simulink model "power_acvoltage"  (Simulink 6.0)
settings: Solver=VariableStepDiscrete  SolverMode=SingleTasking  StartTime=0.0  StopTime=888  MaxStep=1e-03  RelTol=1e-3  AbsTol=1e-6
libraries: powerlib x4
settings Model: Creator=patrice  LastModifiedBy=batserve  ExtModeTrigMode=oneshot  ExtModeArmWhenConnect=off  ExtModeAutoUpdateStatusClock=off
settings DataIOCC: LimitDataPoints=off  SignalLoggingName=sigsOut
settings OptimizationCC: BooleanDataType=off
settings DebuggingCC: SolverPrmCheckMsg=none
settings HardwareCC: TargetUnknown=on
settings RTWCC: TemplateMakefile=grt_unix.tmf

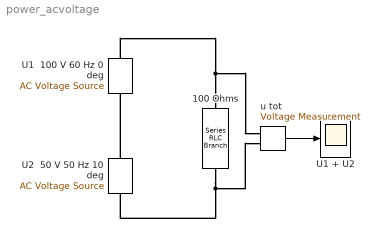
== system power_acvoltage ==
  100 Ohms : powerlib/Elements/Series RLC Branch  Orientation=down  PhysicalDomain=powersysdomain  SubClassName=unknown  PortType=p1  LConnTagsString=__new0  RConnTagsString=__new0  Resistance=100  Inductance=0  Capacitance=inf  Measurements=None
  U1  100 V 60 Hz 0 deg : powerlib/Electrical Sources/AC Voltage Source  Description=source block  Orientation=up  Amplitude=100  Phase=0  Frequency=60  SampleTime=0  Measurements=None
      settings: AttributesFormatString=\n
  U1 + U2 : Scope
      settings: TickLabels=on  TimeRange=0.5  YMin=-180  YMax=180  DataFormat=Array
  U2  50 V 50 Hz 10 deg : powerlib/Electrical Sources/AC Voltage Source  Description=source block  Orientation=up  Amplitude=50  Phase=10  Frequency=50  SampleTime=0  Measurements=None
      settings: AttributesFormatString=\n
  u tot : powerlib/Measurements/Voltage Measurement  Tag=PoWeRsYsTeMmEaSuReMeNt  PhasorSimulation=off  OutputType=Magnitude  PSBequivalent=0
  wires:
  u tot/1 -> U1 + U2/1
  connections:
  U2  50 V 50 Hz 10 deg/RConn1 -- U1  100 V 60 Hz 0 deg/LConn1
  100 Ohms/RConn1 -- U2  50 V 50 Hz 10 deg/LConn1 -- u tot/LConn2
  U1  100 V 60 Hz 0 deg/RConn1 -- 100 Ohms/LConn1 -- u tot/LConn1
